simulink model "CAVE_MachE_sil_test"  (R2019b)
settings: configuration reference "ConfigSetDesktopFixedStep" (kept outside this file)
PreLoadFcn:
  | VSS_BICYCLE=Simulink.Variant('Dual=0');
  | VSS_DUAL=Simulink.Variant('Dual=1');
  | Dual=1;
  | load('DriveCycle2.mat')
PostLoadFcn:
  | if any(exist('dsrtsu_mdlpostloadfcn', 'file') ~= 0), dsrtsu_mdlpostloadfcn('Execute', bdroot); end
InitFcn:
  | , if any(exist('dsmpb_private', 'file') ~= 0), dsmpb_private('dsmpb_mdlclblib', 'Init', bdroot); end,
  | load('DriveCycle2.mat')
model workspace (MAT data in the model file):
  Gas = 0.383333333333
undefined symbols (not defined in the file or in its folder): AccelCmd, ActTqLF_Nm_, ActTqLR_Nm_, ActTqRF_Nm_, ActTqRR_Nm_, BattChargeLimitMaxPwr, BattChargeLimitSocBpts, BattChargeLimitTbl, BattChrgCapcty, BattDischargeLimitSocBpts, BattDischargeLimitTbl, BattDischargeMaxPwr, BattNumCellsParallel, BattNumCellsSeries, BattOpenVoltCapBpts, BattOpenVoltTbl, BattResistSocBpts, BattResistTbl, BattResistTempBpts, BrakeMaxPrs, BrakeMaxTrq, ChassisDistCg2FrontAxle, ChassisDistCg2RearAxle, ChassisVehMass, CltchCmd, CoastDown, DecelCmd, DiffRatio, DiscIntNeverNeededParam, EnvGravCnst, EnvPrs, EnvTemp, FuelSpecificGrav, GearCmd, h, InitStates, lgSw, limitedMCT, MCT, MtrEffSpdBpts, MtrEffTbl, MtrEffTrqBpts, MtrPwrMax, MtrTrqMax, pMCT, SteeringCmd, SupvsryCtrlRegenBrkCutOffTbl, SupvsryCtrlRegenSpdBpts, TestScnrioCycleNum, US06, VEH
libraries: VSIGenLib x39, simulink x27, etargetslib x24, CarMaker4SL x8, vehdynlibtire x8, vehdynlibsuspension x7, vehdynlibtirecommon x7, autolibutils x5, autolibshared x5, VsrLibWheel x4, sharedtransform x3, autolibbatterycommon x2
(part 3 of 11)

== system CAVE_MachE_sil_test/Vehicle Under Test/Vehicle/Rototest and ORNL Interface/RotoTrqPreprocess ==
  AxleTrqRaw : Inport
  Bus Selector1 : BusSelector  OutputSignals=ActTqLF_Nm_,ActTqRF_Nm_,ActTqLR_Nm_,ActTqRR_Nm_
  Compare To Constant : simulink/Logic and Bit Operations/Compare To Constant  relop=>=  const=-15  OutDataTypeStr=boolean
  Compare To Constant1 : simulink/Logic and Bit Operations/Compare To Constant  relop=<=  const=0  OutDataTypeStr=boolean
  Data Type Conversion{1..4} (4 alike) : DataTypeConversion  OutDataTypeStr=double
  FirstOrderFilterTau{,1..3} (4 alike) : VSIGenLib/FirstOrderFilterTau  SystemSampleTime=-1  Latency=0  AutoFrameSizeCalculation=off
  Ground : Ground
  Logical Operator : Logic  AllPortsSameDT=off  OutDataTypeStr=boolean
  ManualTrq_Nm : Constant  Value=0
  Mux : Mux
  Mux1 : Mux
  SatTrq : Saturate  UpperLimit=1000  LowerLimit=-1000
  Tau : Constant  Value=0.01
  TorqueIn : Switch  Criteria=u2 > Threshold
  "TorqueIn " : Switch  Criteria=u2 > Threshold
  AxleTrqRoto : Outport
  AxleTrqVeh : Outport  Port=2
  wires:
  Mux/1 -> AxleTrqRoto/1, TorqueIn/1
  ManualTrq_Nm/1 -> Mux1/4, Mux1/3, Mux1/2, Mux1/1
  Tau/1 -> FirstOrderFilterTau/2, FirstOrderFilterTau1/2, FirstOrderFilterTau2/2, FirstOrderFilterTau3/2
  Ground/1 -> "TorqueIn "/1
  Logical Operator/1 -> "TorqueIn "/2
  Data Type Conversion4/1 -> Mux/4  "RR"
  Data Type Conversion3/1 -> Mux/3  "LR"
  Mux1/1 -> TorqueIn/3
  [Switch] -> TorqueIn/2
  Bus Selector1/4 -> FirstOrderFilterTau3/1  "<ActTqRR_Nm_>"
  Compare To Constant/1 -> Logical Operator/1
  Bus Selector1/3 -> FirstOrderFilterTau2/1  "<ActTqLR_Nm_>"
  Bus Selector1/2 -> FirstOrderFilterTau1/1  "<ActTqRF_Nm_>"
  TorqueIn/1 -> SatTrq/1
  "TorqueIn "/1 -> AxleTrqVeh/1  "Trq"
  FirstOrderFilterTau1/1 -> Data Type Conversion2/1
  Data Type Conversion2/1 -> Mux/2  "RF"
  AxleTrqRaw/1 -> Bus Selector1/1
  FirstOrderFilterTau/1 -> Data Type Conversion1/1
  FirstOrderFilterTau3/1 -> Data Type Conversion4/1
  Bus Selector1/1 -> FirstOrderFilterTau/1  "<ActTqLF_Nm_>"
  Compare To Constant1/1 -> Logical Operator/2
  SatTrq/1 -> "TorqueIn "/3, Compare To Constant1/1, Compare To Constant/1
  FirstOrderFilterTau2/1 -> Data Type Conversion3/1
  Data Type Conversion1/1 -> Mux/1  "LF"

== system CAVE_MachE_sil_test/Vehicle Under Test/Vehicle/Rototest and ORNL Interface/Subsystem2 ==
  AxlTorq : Inport
  BusCreator1 : BusCreator  Inputs=16
  BusCreator2 : BusCreator  Inputs=16
  Constant : Constant  Value=0
  Constant1 : Constant  Value=0
  Demux : Demux  Outputs=16
  Terminator : Terminator
  Zero1 : Constant  Value=0
  Zero2 : Constant  Value=0
  Zero5 : Constant  Value=0
  BrakeUpd : Outport
  wires:
  Demux/9 -> BusCreator1/9  "Brake IF Trq_Reg_trg FL"
  Demux/6 -> BusCreator1/6  "Brake IF Trq_PB FR"
  Constant1/1 -> BusCreator2/1, BusCreator2/2  "Brake IF Trq_WB FL"
  Demux/14 -> BusCreator1/14  "Brake IF Trq_DriveSrc_trg d1"
  Zero2/1 -> BusCreator2/16, BusCreator2/15, BusCreator2/14, BusCreator2/13  "Brake IF Trq_DriveSrc_trg d3"
  Demux/11 -> BusCreator1/11  "Brake IF Trq_Reg_trg RL"
  Demux/15 -> BusCreator1/15  "Brake IF Trq_DriveSrc_trg d2"
  Demux/2 -> BusCreator1/2  "Brake IF Trq_WB FR"
  Demux/16 -> BusCreator1/16  "Brake IF Trq_DriveSrc_trg d3"
  Zero1/1 -> BusCreator2/12, BusCreator2/11, BusCreator2/10, BusCreator2/9  "Brake IF Trq_Reg_trg RR"
  Demux/4 -> BusCreator1/4  "Brake IF Trq_WB RR"
  Demux/3 -> BusCreator1/3  "Brake IF Trq_WB RL"
  Constant/1 -> BusCreator2/4, BusCreator2/3  "Brake IF Trq_WB RL"
  BusCreator1/1 -> BrakeUpd/1
  Demux/1 -> BusCreator1/1  "Brake IF Trq_WB FL"
  Demux/8 -> BusCreator1/8  "Brake IF Trq_PB RR"
  Demux/10 -> BusCreator1/10  "Brake IF Trq_Reg_trg FR"
  BusCreator2/1 -> Demux/1
  Demux/13 -> BusCreator1/13  "Brake IF Trq_DriveSrc_trg d0"
  Demux/5 -> BusCreator1/5  "Brake IF Trq_PB FL"
  Demux/7 -> BusCreator1/7  "Brake IF Trq_PB RL"
  Zero5/1 -> BusCreator2/8, BusCreator2/7, BusCreator2/6, BusCreator2/5  "Brake IF Trq_PB RR"
  Demux/12 -> BusCreator1/12  "Brake IF Trq_Reg_trg RR"
  AxlTorq/1 -> Terminator/1

== system CAVE_MachE_sil_test/Vehicle Under Test/Vehicle/Rototest and ORNL Interface/To Rototest with Band-Aid ==
  note: Torque Model: Low speed
      | Speed Model: Normal speed
  note: OutMode = 0 is Torque
      | OutMode = 1 is Speed
  note: Switch = 0 Overides
      | Switch = 1 Model
  SpeedCmd_rps : Inport
  AxleTrq_roto_Nm : Inport  Port=2
  BRAKE_PRESSED : Inport  Port=3
  Vehicle_Speed_kph : Inport  Port=4
  Band-Aid : Subsystem
  Demux : Demux
  Demux1 : Demux
  Demux2 : Demux
  Logging : Subsystem  Commented=on
  MasterSw : Constant
  Mode Override : Subsystem
  ModeOut : Switch  Criteria=u2 > Threshold
  ModeSwitch : MultiPortSwitch  DataPortOrder=Zero-based contiguous  Inputs=2  zeroidx=on
  Mux2 : Mux
  Mux4 : Mux
  Mux5 : Mux
  RateLimSpd : RateLimiter  RisingSlewLimit=500  FallingSlewLimit=-500  SampleTimeMode=inherited
  RotoTestEthTx : Subsystem  AncestorBlock=VSIGenLib/RotoTestEthTx
      mask Display:
      | color('white')
      | disp('RotTestEthTx')
      | port_label('input', 1, 'RefLF_NmORrpm')
      | port_label('input', 2, 'RefRF_NmORrpm')
      | port_label('input', 3, 'RefLR_NmORrpm')
      | port_label('input', 4, 'RefRR_NmORrpm')
      | port_label('input', 5, 'SqTrRR')
      | port_label('input', 6, 'SqTrLR')
      | port_label('input', 7, 'SqTrRF')
      | port_label('input', 8, 'SqTrLF')
      | port_label('input', 9, 'SystemActive')
      | port_label('output', 1, 'Status (bool)')
      | port_label('output', 2, 'Sent Bytes (int)')
  SatSpd : Saturate  UpperLimit=700  LowerLimit=0
  Scope : Scope
  Scope1 : Scope
  SpeedOut : Switch  Criteria=u2 > Threshold
  SystemActive : Constant  Value=0  OutDataTypeStr=uint8
  TrqSpd Override : Subsystem
  ZeroTorque : Constant  Value=0  OutDataTypeStr=uint8
  rads2rpm : Gain  Gain=9.5492965964254
  Out1 : Outport
  tag scope: Switch=global
  wires:
  Mux4/1 -> ModeSwitch/2
  Demux/3 -> Mux2/3  "LRIn"
  Demux1/4 -> RotoTestEthTx/4(RefRR_NmORrpm)
  Demux/2 -> Mux2/2  "RFIn"
  MasterSw/1 -> [Switch]
  TrqSpd Override/1(Ovr) -> SpeedOut/3
  ZeroTorque/1 -> Mux4/2, Mux4/3, Mux4/4, Mux4/1
  Demux/1 -> Mux2/1  "LFIn"
  SpeedOut/1 -> RateLimSpd/1
  RateLimSpd/1 -> SatSpd/1
  rads2rpm/1 -> Demux/1
  ModeSwitch/1 -> Demux1/1
  Demux/4 -> Mux2/4  "RRIn"
  Band-Aid/1(OutMode) -> Mux5/4, Mux5/3, Mux5/2, Mux5/1, ModeSwitch/1
  ModeOut/1 -> Demux2/1
  [Switch] -> SpeedOut/2
  SatSpd/1 -> Scope1/1, ModeSwitch/3  "Spd"
  [Switch] -> ModeOut/2
  Mux5/1 -> ModeOut/1
  Demux2/1 -> RotoTestEthTx/5(SpTqRR)
  Demux1/3 -> RotoTestEthTx/3(RefLR_NmORrpm)
  Demux2/3 -> RotoTestEthTx/7(SpTqRF)
  Demux2/2 -> RotoTestEthTx/6(SpTqLR)
  SystemActive/1 -> RotoTestEthTx/9(SystemActive)
  RotoTestEthTx/1(Output) -> Out1/1  "ByteSend"
  Demux1/1 -> Scope/1, RotoTestEthTx/1(RefLF_NmORrpm)
  Demux1/2 -> RotoTestEthTx/2(RefRF_NmORrpm)
  Demux2/4 -> RotoTestEthTx/8(SpTqLF)
  SpeedCmd_rps/1 -> rads2rpm/1
  Mode Override/1(Ovr) -> ModeOut/3
  AxleTrq_roto_Nm/1 -> Band-Aid/2(InTrq_Nm)
  Mux2/1 -> Band-Aid/1(InSpd_rpm)
  Band-Aid/2(OutSpd_rpm) -> SpeedOut/1
  BRAKE_PRESSED/1 -> Band-Aid/3(BRAKE_PRESSED)
  Vehicle_Speed_kph/1 -> Band-Aid/4(VehSpd_kph)

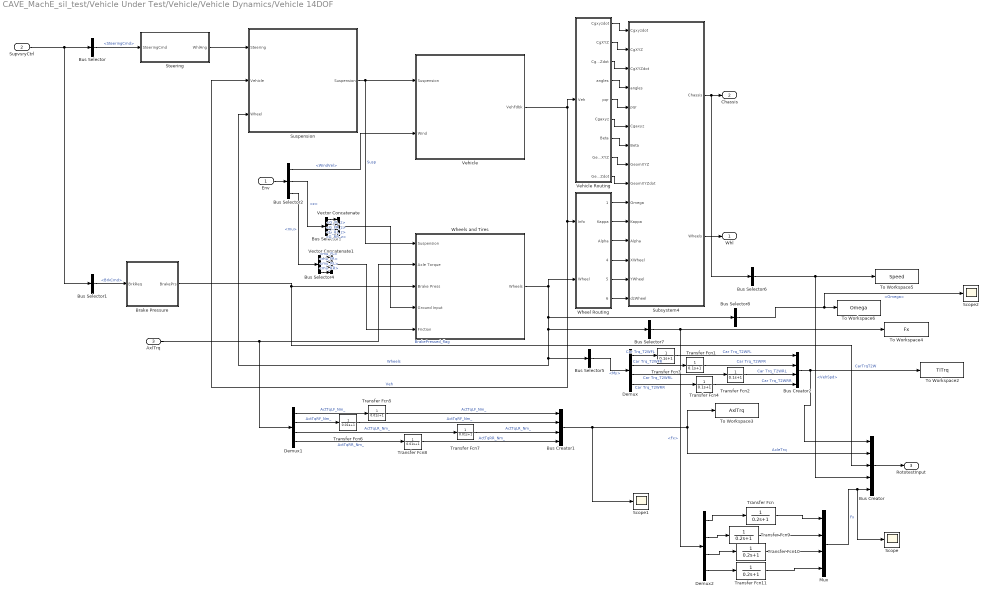
== system CAVE_MachE_sil_test/Vehicle Under Test/Vehicle/Vehicle Dynamics/Vehicle 14DOF ==
  Env : Inport
  SupvsryCtrl : Inport  Port=2
  AxlTrq : Inport  Port=3
  Brake Pressure : Subsystem
  Bus Creator : BusCreator  Inputs=5
  Bus Creator1 : BusCreator  Inputs=ActTqLF_Nm_,ActTqRF_Nm_,ActTqLR_Nm_,ActTqRR_Nm_
  Bus Creator2 : BusCreator  Inputs=Car Trq_T2WFL,Car Trq_T2WFR,Car Trq_T2WRL,Car Trq_T2WRR
  Bus Selector : BusSelector  OutputSignals=SteeringCmd
  Bus Selector1 : BusSelector  OutputSignals=BrkCmd
  Bus Selector2 : BusSelector  OutputSignals=WindVel,GndBus.z,GndBus.mu
  Bus Selector3 : BusSelector  OutputSignals=G_FL_z,G_FR_z,G_RL_z,G_RR_z
  Bus Selector4 : BusSelector  OutputSignals=mu_FL,mu_FR,mu_RL,mu_RR
  Bus Selector5 : BusSelector  OutputSignals=TireFrame.My
  Bus Selector6 : BusSelector  OutputSignals=VehSpd
  Bus Selector7 : BusSelector  OutputSignals=TireFrame.Fx
  Bus Selector8 : BusSelector  OutputSignals=TireFrame.Omega
  Demux : Demux
  Demux1 : Demux
  Demux2 : Demux
  Mux : Mux
  Scope : Scope
  Scope1 : Scope
  Scope2 : Scope
  Steering : Subsystem
  Subsystem4 : Subsystem
  Suspension : Subsystem  VariantControlMode=Label  Variant=on  LabelModeActiveChoice=3
      mask Display:
      | switch str2num(get_param(gcb,'ActiveVariant'))
      |     case 1
      |         image('suspdw.png');
      |     case 2
      |         image([imread('suspindmap.png');imread('suspsamap.png')]);
      |     case 3
      |          image([imread('suspmacp.png');imread('suspsacoil.png')]);
      |     case 4
      |          image('suspmacp.png');
      |     case 5
      |          image('suspindmap.png');
      | end
  To Workspace2 : ToWorkspace  VariableName=TiTrq  SampleTime=-1
      settings: Save2DSignal=2-D array (concatenate along first dimension)
  To Workspace3 : ToWorkspace  VariableName=AxlTrq  SampleTime=-1
      settings: Save2DSignal=2-D array (concatenate along first dimension)
  To Workspace4 : ToWorkspace  VariableName=Fx  SampleTime=-1
      settings: Save2DSignal=2-D array (concatenate along first dimension)
  To Workspace5 : ToWorkspace  VariableName=Speed  SampleTime=-1
      settings: Save2DSignal=2-D array (concatenate along first dimension)
  To Workspace6 : ToWorkspace  VariableName=Omega  SampleTime=-1
      settings: Save2DSignal=2-D array (concatenate along first dimension)
  Transfer Fcn{,9..11} (4 alike) : TransferFcn  Denominator=[0.2 1]
  Transfer Fcn{1..4} (4 alike) : TransferFcn  Denominator=[0.1 1]
  Transfer Fcn{5..8} (4 alike) : TransferFcn  Denominator=[0.01 1]
  Vector Concatenate : Concatenate  NumInputs=4
  Vector Concatenate1 : Concatenate  NumInputs=4
  Vehicle : Subsystem
      mask Display: image('6dofcar.png');
  Vehicle Routing : Subsystem
  Wheel Routing : Subsystem
  Wheels and Tires : Subsystem
      mask Display: image('wheel3dof.png')
  Whl : Outport
  Chassis : Outport  Port=2
  RototestInput : Outport  Port=3
  wires:
  Vehicle Routing/9(GeomXYZdot) -> Subsystem4/9(GeomXYZdot)
  Vehicle Routing/8(GeomXYZ) -> Subsystem4/8(GeomXYZ)
  Vehicle Routing/1(Cgxyzdot) -> Subsystem4/1(Cgxyzdot)
  Vehicle Routing/5(pqr) -> Subsystem4/5(pqr)
  Vehicle Routing/4(angles) -> Subsystem4/4(angles)
  Vehicle Routing/3(CgXYZdot) -> Subsystem4/3(CgXYZdot)
  Vehicle Routing/7(Beta) -> Subsystem4/7(Beta)
  Wheels and Tires/1(Wheels) -> Wheel Routing/2(Wheel), Bus Selector7/1, Bus Selector5/1, Suspension/3(Wheel), Bus Selector8/1  "Wheels"
  Vehicle Routing/2(CgXYZ) -> Subsystem4/2(CgXYZ)
  Vehicle/1(VehFdbk) -> Suspension/2(Vehicle), Wheel Routing/1(Info), Vehicle Routing/1(Veh)  "Veh"
  Suspension/1(Suspension) -> Vehicle/1(Suspension), Wheels and Tires/1(Suspension)  "Susp"
  Bus Selector2/1 -> Vehicle/2(Wind)  "<WindVel>"
  Steering/1(WhlAng) -> Suspension/1(Steering)
  Bus Selector/1 -> Steering/1(SteeringCmd)  "<SteeringCmd>"
  SupvsryCtrl/1 -> Bus Selector/1, Bus Selector1/1
  Bus Selector1/1 -> Brake Pressure/1(BrkReq)  "<BrkCmd>"
  Env/1 -> Bus Selector2/1
  Vehicle Routing/6(Cgaxyz) -> Subsystem4/6(Cgaxyz)
  Wheel Routing/1(Omega) -> Subsystem4/10(Omega)
  Wheel Routing/3(Alpha) -> Subsystem4/12(Alpha)
  Wheel Routing/4(XWheel) -> Subsystem4/13(XWheel)
  Wheel Routing/2(Kappa) -> Subsystem4/11(Kappa)
  Wheel Routing/5(YWheel) -> Subsystem4/14(YWheel)
  Wheel Routing/6(ZWheel) -> Subsystem4/15(dzWheel)
  Subsystem4/2(Wheels) -> Whl/1
  AxlTrq/1 -> Demux1/1, Wheels and Tires/2(Axle Torque)
  Bus Selector2/2 -> Bus Selector3/1  "<z>"
  Bus Selector3/1 -> Vector Concatenate/1  "<G_FL_z>"
  Bus Selector3/2 -> Vector Concatenate/2  "<G_FR_z>"
  Bus Selector3/3 -> Vector Concatenate/3  "<G_RL_z>"
  Bus Selector3/4 -> Vector Concatenate/4  "<G_RR_z>"
  Vector Concatenate/1 -> Wheels and Tires/4(Ground Input)
  Bus Selector4/4 -> Vector Concatenate1/4  "<mu_RR>"
  Bus Selector2/3 -> Bus Selector4/1  "<mu>"
  Bus Selector4/3 -> Vector Concatenate1/3  "<mu_RL>"
  Bus Selector4/2 -> Vector Concatenate1/2  "<mu_FR>"
  Bus Selector4/1 -> Vector Concatenate1/1  "<mu_FL>"
  Vector Concatenate1/1 -> Wheels and Tires/5(Friction)
  Demux/3 -> Transfer Fcn2/1  "Car Trq_T2WRL"
  Bus Selector6/1 -> Bus Creator/4, To Workspace5/1  "<VehSpd>"
  Brake Pressure/1(BrakePrs) -> Bus Creator/3, Wheels and Tires/3(Brake Press)  "BrakePressed_flag"
  Demux/2 -> Transfer Fcn1/1  "Car Trq_T2WFR"
  Demux1/1 -> Transfer Fcn5/1  "ActTqLF_Nm_"
  Demux1/4 -> Transfer Fcn8/1  "ActTqRR_Nm_"
  Demux1/3 -> Transfer Fcn7/1  "ActTqLR_Nm_"
  Demux/4 -> Transfer Fcn4/1  "Car Trq_T2WRR"
  Bus Creator1/1 -> Scope1/1, Bus Creator/2, To Workspace3/1  "AxleTrq"
  Demux1/2 -> Transfer Fcn6/1  "ActTqRF_Nm_"
  Bus Creator2/1 -> Bus Creator/1, To Workspace2/1  "CarTrqT2W"
  Demux/1 -> Transfer Fcn3/1  "Car Trq_T2WFL"
  Bus Selector5/1 -> Demux/1  "<My>"
  Subsystem4/1(Chassis) -> Bus Selector6/1, Chassis/1
  Bus Selector7/1 -> Demux2/1, To Workspace4/1  "<Fx>"
  Bus Selector8/1 -> Scope2/1, To Workspace6/1  "<Omega>"
  Bus Creator/1 -> RototestInput/1
  Transfer Fcn3/1 -> Bus Creator2/1  "Car Trq_T2WFL"
  Transfer Fcn1/1 -> Bus Creator2/2  "Car Trq_T2WFR"
  Transfer Fcn2/1 -> Bus Creator2/3  "Car Trq_T2WRL"
  Transfer Fcn4/1 -> Bus Creator2/4  "Car Trq_T2WRR"
  Transfer Fcn5/1 -> Bus Creator1/1  "ActTqLF_Nm_"
  Transfer Fcn6/1 -> Bus Creator1/2  "ActTqRF_Nm_"
  Transfer Fcn7/1 -> Bus Creator1/3  "ActTqLR_Nm_"
  Transfer Fcn8/1 -> Bus Creator1/4  "ActTqRR_Nm_"
  Demux2/1 -> Transfer Fcn/1
  Transfer Fcn/1 -> Mux/1
  Demux2/2 -> Transfer Fcn9/1
  Transfer Fcn9/1 -> Mux/2
  Demux2/3 -> Transfer Fcn10/1
  Demux2/4 -> Transfer Fcn11/1
  Transfer Fcn10/1 -> Mux/3
  Transfer Fcn11/1 -> Mux/4
  Mux/1 -> Scope/1, Bus Creator/5  "Fx"

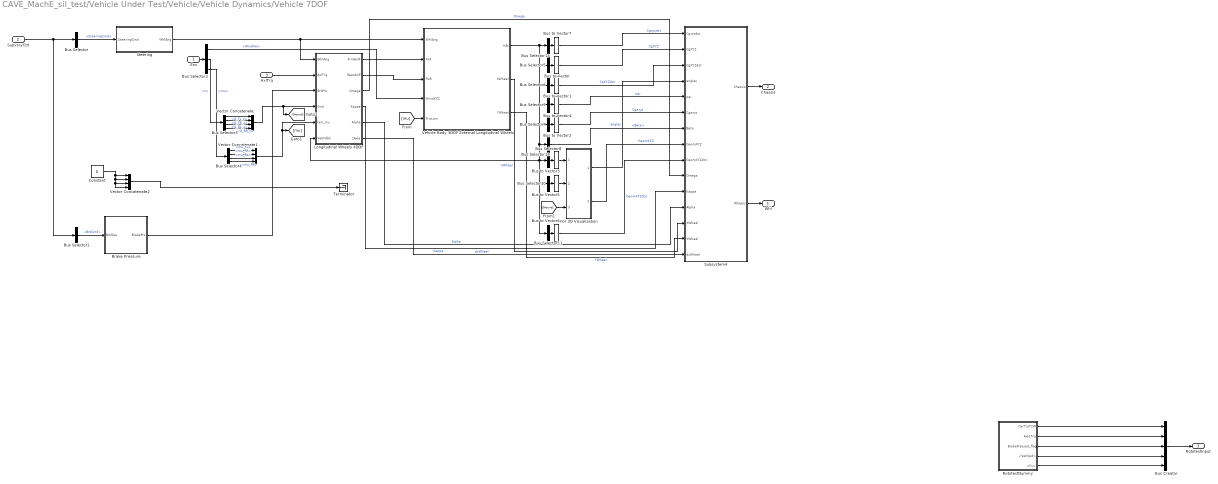
== system CAVE_MachE_sil_test/Vehicle Under Test/Vehicle/Vehicle Dynamics/Vehicle 7DOF ==
  Env : Inport
  SupvsryCtrl : Inport  Port=2
  AxlTrq : Inport  Port=3
  Brake Pressure : Subsystem
  Bus Creator : BusCreator  Inputs=5
  Bus Selector : BusSelector  OutputSignals=SteeringCmd
  Bus Selector1 : BusSelector  OutputSignals=BrkCmd
  Bus Selector10 : BusSelector  OutputSignals=InertFrm.Geom.Disp.X,InertFrm.Geom.Disp.Y,InertFrm.Geom.Disp.Z  OutputAsBus=on
  Bus Selector11 : BusSelector  OutputSignals=InertFrm.Geom.Vel.Xdot,InertFrm.Geom.Vel.Ydot,InertFrm.Geom.Vel.Zdot  OutputAsBus=on
  Bus Selector12 : BusSelector  OutputSignals=BdyFrm.Geom.Ang.Beta
  Bus Selector13 : BusSelector  OutputSignals=BdyFrm.Cg.Vel.xdot,BdyFrm.Cg.Vel.ydot,BdyFrm.Cg.Vel.zdot  OutputAsBus=on
  Bus Selector2 : BusSelector  OutputSignals=WindVel,GndBus.z,GndBus.mu
  Bus Selector3 : BusSelector  OutputSignals=G_FL_z,G_FR_z,G_RL_z,G_RR_z
  Bus Selector4 : BusSelector  OutputSignals=mu_FL,mu_FR,mu_RL,mu_RR
  Bus Selector5 : BusSelector  OutputSignals=InertFrm.Cg.Disp.X,InertFrm.Cg.Disp.Y,InertFrm.Cg.Disp.Z  OutputAsBus=on
  Bus Selector6 : BusSelector  OutputSignals=InertFrm.Cg.Vel.Xdot,InertFrm.Cg.Vel.Ydot,InertFrm.Cg.Vel.Zdot  OutputAsBus=on
  Bus Selector7 : BusSelector  OutputSignals=BdyFrm.Cg.Acc.ax,BdyFrm.Cg.Acc.ay,BdyFrm.Cg.Acc.az  OutputAsBus=on
  Bus Selector8 : BusSelector  OutputSignals=InertFrm.Cg.Ang.phi,InertFrm.Cg.Ang.theta,InertFrm.Cg.Ang.psi  OutputAsBus=on
  Bus Selector9 : BusSelector  OutputSignals=BdyFrm.Cg.AngVel.p,BdyFrm.Cg.AngVel.q,BdyFrm.Cg.AngVel.r  OutputAsBus=on
  Bus to Vector{,1..7} (8 alike) : BusToVector
  Constant : Constant  Value=0
  For 3D Visualization : MATLAB Function  TreatAsAtomicUnit=on  mask{trackW=1.9, wheelB=ChassisDistCg2FrontAxle+ChassisDistCg2RearAxle}
      mask prompts: trackW "Vehicle track width, trackW [m]:"; wheelB "Vehicle wheelbase, wheelB [m]:"
      mask help: This block converts wheel ground height information into estimates of vehicle pitch, roll angles and vertical height in order to help in the visualization 3DOF based simulations with changes in terrain. Note that the resulting signals are only used as a visualization aid and do not account for the physical affects of the vehicle interacting with variable terrain or changes in orientation.
  Longitudinal Wheels 4DOF : Subsystem  VariantControl=1
      settings: AttributesFormatString=%<wheelMode>
  RototestDummy : Subsystem
  Steering : Subsystem
  Subsystem4 : Subsystem
  Terminator : Terminator
  Vector Concatenate : Concatenate  NumInputs=4
  Vector Concatenate1 : Concatenate  NumInputs=4
  Vector Concatenate2 : Concatenate  NumInputs=4
  Vehicle Body 3DOF External Longitudinal Wheels : Subsystem  VariantControlMode=Label  Variant=on  VariantControl=Variant1  LabelModeActiveChoice=1
      settings: AttributesFormatString=%<trackMode>
  Whl : Outport
  Chassis : Outport  Port=2
  RototestInput : Outport  Port=3
  wires:
  Bus Selector2/1 -> Vehicle Body 3DOF External Longitudinal Wheels/4(WindXYZ)  "<WindVel>"
  Bus Selector/1 -> Steering/1(SteeringCmd)  "<SteeringCmd>"
  SupvsryCtrl/1 -> Bus Selector/1, Bus Selector1/1
  Bus Selector1/1 -> Brake Pressure/1(BrkReq)  "<BrkCmd>"
  Env/1 -> Bus Selector2/1
  Subsystem4/2(Wheels) -> Whl/1
  Subsystem4/1(Chassis) -> Chassis/1
  Bus Selector2/2 -> Bus Selector3/1  "<z>"
  Bus Selector3/1 -> Vector Concatenate/1  "<G_FL_z>"
  Bus Selector3/2 -> Vector Concatenate/2  "<G_FR_z>"
  Bus Selector3/3 -> Vector Concatenate/3  "<G_RL_z>"
  Bus Selector3/4 -> Vector Concatenate/4  "<G_RR_z>"
  Bus Selector4/4 -> Vector Concatenate1/4  "<mu_RR>"
  Bus Selector2/3 -> Bus Selector4/1  "<mu>"
  Bus Selector4/3 -> Vector Concatenate1/3  "<mu_RL>"
  Bus Selector4/2 -> Vector Concatenate1/2  "<mu_FR>"
  Bus Selector4/1 -> Vector Concatenate1/1  "<mu_FL>"
  Vector Concatenate2/1 -> Terminator/1
  Constant/1 -> Vector Concatenate2/4, Vector Concatenate2/3, Vector Concatenate2/2, Vector Concatenate2/1
  Bus to Vector2/1 -> Subsystem4/6(Cgaxyz)  "Cgaxyz"
  Bus Selector8/1 -> Bus to Vector3/1
  Bus to Vector5/1 -> For 3D Visualization/2(GemoXYZIn)
  Bus Selector12/1 -> Subsystem4/7(Beta)  "<Beta>"
  Bus Selector5/1 -> Bus to Vector/1
  For 3D Visualization/1(angles) -> Subsystem4/4(angles)  "angles"
  For 3D Visualization/2(GeomXYZ) -> Subsystem4/8(GeomXYZ)  "GeomXYZ"
  Bus to Vector6/1 -> Subsystem4/9(GeomXYZdot)  "GeomXYZdot"
  Bus Selector13/1 -> Bus to Vector7/1
  Bus to Vector7/1 -> Subsystem4/1(Cgxyzdot)  "Cgxyzdot"
  Bus Selector10/1 -> Bus to Vector5/1
  Longitudinal Wheels 4DOF/1(FrntAxlF) -> Vehicle Body 3DOF External Longitudinal Wheels/2("FwF ")
  Bus Selector11/1 -> Bus to Vector6/1
  Bus Selector9/1 -> Bus to Vector4/1
  [mu] -> Vehicle Body 3DOF External Longitudinal Wheels/5(Friction)
  Longitudinal Wheels 4DOF/2(RearAxlF) -> Vehicle Body 3DOF External Longitudinal Wheels/3("FwR ")
  Bus to Vector4/1 -> Subsystem4/5(pqr)  "pqr"
  Vehicle Body 3DOF External Longitudinal Wheels/3(" YWheel") -> Subsystem4/14(YWheel)  "YWheel"
  Vector Concatenate/1 -> Longitudinal Wheels 4DOF/4(Gnd), [Ground]
  Bus to Vector/1 -> Subsystem4/2(CgXYZ)  "CgXYZ"
  AxlTrq/1 -> Longitudinal Wheels 4DOF/2(AxlTrq)
  Vehicle Body 3DOF External Longitudinal Wheels/1(" Info") -> Bus Selector13/1, Bus Selector11/1, Bus Selector10/1, Longitudinal Wheels 4DOF/6(VehFdbk), Bus Selector8/1, Bus Selector12/1, Bus Selector7/1, Bus Selector9/1, Bus Selector6/1, Bus Selector5/1
  [Ground] -> For 3D Visualization/3(GroundZ)
  Bus to Vector1/1 -> Subsystem4/3(CgXYZdot)  "CgXYZdot"
  Bus to Vector3/1 -> For 3D Visualization/1(angleIn)
  Longitudinal Wheels 4DOF/5(Alpha) -> Subsystem4/12(Alpha)  "Alpha"
  Vector Concatenate1/1 -> Longitudinal Wheels 4DOF/5(lam_mu), [mu]
  Bus Selector6/1 -> Bus to Vector1/1
  Brake Pressure/1(BrakePrs) -> Longitudinal Wheels 4DOF/3(BrkPrs)
  Vehicle Body 3DOF External Longitudinal Wheels/2(" XWheel") -> Subsystem4/13(XWheel)  "XWheel"
  Longitudinal Wheels 4DOF/4(Kappa) -> Subsystem4/11(Kappa)  "Kappa"
  Steering/1(WhlAng) -> Longitudinal Wheels 4DOF/1(WhlAng), Vehicle Body 3DOF External Longitudinal Wheels/1(WhlAng)
  Longitudinal Wheels 4DOF/6(zAxle) -> Subsystem4/15(dzWheel)  "dzWheel"
  Bus Selector7/1 -> Bus to Vector2/1
  Longitudinal Wheels 4DOF/3(Omega) -> Subsystem4/10(Omega)  "Omega"
  Bus Creator/1 -> RototestInput/1
  RototestDummy/1(CarTrqT2W) -> Bus Creator/1
  RototestDummy/2(AxleTrq) -> Bus Creator/2
  RototestDummy/3(BrakePressed_flag) -> Bus Creator/3
  RototestDummy/4(<VehSpd>) -> Bus Creator/4
  RototestDummy/5(<Fx>) -> Bus Creator/5

== system CAVE_MachE_sil_test/Vehicle Under Test/Vehicle/Vehicle Dynamics/Vehicle Longitudinal ==
  Env : Inport
  SupvsryCtrl : Inport  Port=2
  AxlTrq : Inport  Port=3
  Brake Pressure : Subsystem
  Bus Creator : BusCreator  Inputs=5
  Bus Selector1 : BusSelector  OutputSignals=BrkCmd
  Bus Selector2 : BusSelector  OutputSignals=RoadGrade,WindVel,GndBus.z,GndBus.mu
  Bus Selector3 : BusSelector  OutputSignals=G_FL_z,G_FR_z,G_RL_z,G_RR_z
  Bus Selector4 : BusSelector  OutputSignals=mu_FL,mu_FR,mu_RL,mu_RR
  Constant : Constant  Value=0
  Longitudinal Wheels : Subsystem  AncestorBlock=LibWheels/Longitudinal Wheels and Brakes
  RototestDummy : Subsystem
  Selector : Selector  InputPortWidth=3  IndexOptions=Index vector (dialog)  Indices=1  OutputSizes=1
  Terminator : Terminator
  Terminator1 : Terminator
  Vector Concatenate : Concatenate  NumInputs=4
  Vector Concatenate1 : Concatenate  NumInputs=4
  Vector Concatenate2 : Concatenate  NumInputs=4
  Vehicle Body : Subsystem
  Whl : Outport
  Chassis : Outport  Port=2
  RototestInput : Outport  Port=3
  wires:
  Vehicle Body/1(Chassis) -> Chassis/1
  Longitudinal Wheels/1(Whl) -> Whl/1
  Bus Selector4/1 -> Vector Concatenate1/1  "<mu_FL>"
  Bus Selector2/4 -> Bus Selector4/1  "<mu>"
  Vector Concatenate1/1 -> Terminator1/1
  Brake Pressure/1(BrakePrs) -> Longitudinal Wheels/1(BrkPrs)
  Bus Selector4/2 -> Vector Concatenate1/2  "<mu_FR>"
  Bus Selector3/1 -> Vector Concatenate/1  "<G_FL_z>"
  Bus Selector3/4 -> Vector Concatenate/4  "<G_RR_z>"
  Bus Selector2/3 -> Bus Selector3/1  "<z>"
  Env/1 -> Bus Selector2/1
  Vector Concatenate/1 -> Terminator/1
  Bus Selector4/3 -> Vector Concatenate1/3  "<mu_RL>"
  Bus Selector3/2 -> Vector Concatenate/2  "<G_FR_z>"
  SupvsryCtrl/1 -> Bus Selector1/1
  Constant/1 -> Vector Concatenate2/4, Vector Concatenate2/3, Vector Concatenate2/2, Vector Concatenate2/1
  Bus Selector4/4 -> Vector Concatenate1/4  "<mu_RR>"
  Bus Selector1/1 -> Brake Pressure/1(BrkReq)  "<BrkCmd>"
  Bus Selector3/3 -> Vector Concatenate/3  "<G_RL_z>"
  AxlTrq/1 -> Longitudinal Wheels/2(AxleTorq)
  Bus Selector2/2 -> Selector/1  "<WindVel>"
  Bus Selector2/1 -> Vehicle Body/1(RoadGrade)  "<RoadGrade>"
  Selector/1 -> Vehicle Body/2(WindX)
  Bus Creator/1 -> RototestInput/1
  RototestDummy/5(<Fx>) -> Bus Creator/5
  RototestDummy/4(<VehSpd>) -> Bus Creator/4
  RototestDummy/3(BrakePressed_flag) -> Bus Creator/3
  RototestDummy/2(AxleTrq) -> Bus Creator/2
  RototestDummy/1(CarTrqT2W) -> Bus Creator/1
  connections:
  Longitudinal Wheels/RConn2 -- Vehicle Body/LConn2
  Vehicle Body/LConn1 -- Longitudinal Wheels/RConn1

== system CAVE_MachE_sil_test/Vehicle Under Test/Vehicle/Battery/Battery/Lithium Ion Battery Pack1 ==
  note: Info
  BattCurr : Inport  Unit=A
  BattTemp : Inport  Port=2  Unit=K
  Datasheet Battery Internal : Subsystem  AncestorBlock=autolibbatterycommon/Datasheet Battery Internal
  Info Bus : autolibbatterycommon/Info  RefBlkName='autolibdatasheetbattery/Datasheet Battery'
      settings: SourceProductName=Powertrain Blockset  SourceProductBaseCode=PW
  Output Passthrough : autolibbatterycommon/Output Passthrough  SystemSampleTime=-1  Latency=0  AutoFrameSizeCalculation=off
      settings: SourceProductName=Powertrain Blockset  SourceProductBaseCode=PW
  Info : Outport  VectorParamsAs1DForOutWhenUnconnected=off
  BattVolt : Outport  Port=2  Unit=V  VectorParamsAs1DForOutWhenUnconnected=off
  wires:
  [BattPwrLoss] -> Info Bus/5
  Output Passthrough/1 -> BattVolt/1, [BattVolt]
  [BattVolt] -> Info Bus/4
  Datasheet Battery Internal/1(LdCurrFeed) -> [LdCurrFeed]
  [LdCurrFeed] -> Info Bus/3
  Datasheet Battery Internal/5(BattPwrLoss) -> [BattPwrLoss]
  Datasheet Battery Internal/2(OutVoltUnfilt) -> Output Passthrough/1
  Datasheet Battery Internal/3(LdAmpHr) -> [LdAmpHr]
  Datasheet Battery Internal/4(BattSoc) -> [BattSoc]
  BattTemp/1 -> Datasheet Battery Internal/2(BattTemp)
  BattCurr/1 -> Datasheet Battery Internal/1(BattCurr)
  Info Bus/1 -> Info/1
  [BattSoc] -> Info Bus/2
  [LdAmpHr] -> Info Bus/1

== system CAVE_MachE_sil_test/Vehicle Under Test/Vehicle/Driver and Drive Cycle/Driver and PI with FF Control/Vehicle Speed Controller ==
  note: ToDo: Maybe do something clever with FF and Brake, or maybe not.
      | Bleed FF based on refspd derivative
  RefSpd : Inport
  VehicleSpeed : Inport  Port=2
  Compare To Constant1 : simulink/Logic and Bit Operations/Compare To Constant  relop=<=  const=0.1  OutDataTypeStr=boolean  ZeroCross=off
  Compare To Constant3 : simulink/Logic and Bit Operations/Compare To Constant  relop=<=  const=0  OutDataTypeStr=boolean  ZeroCross=off
  Constant : Constant  Value=0
  Constant1 : Constant  Value=0
  Feedforward : Lookup_n-D  NumberOfTableDimensions=1  BreakpointsForDimension1="[0 10    20    30    40    50    60    70    80    90   100   110   120   130   140   150   160]"  Table="[0\t3.5\t12.5\t16\t20\t21\t22\t24.5\t26\t29.5\t32\t33\t34\t36\t37\t38\t39]"  ExtrapMethod=Clip  InternalRulePriority=Speed  RndMeth=Simplest  InputSameDT=on
  Feedforward1 : Lookup_n-D  NumberOfTableDimensions=1  BreakpointsForDimension1="[0 10    20    30    40    50    60    70    80    90   100   110   120   130   140   150   160]"  Table="[0 2.6021    4.7790    6.8575    8.1555    9.4176   10.7914   12.3245   14.1570   15.9699   17.4605   19.0355   21.3079   22.8407   25.3373   26.9453   28.6975]"  ExtrapMethod=Clip  InternalRulePriority=Speed  RndMeth=Simplest  InputSameDT=on
  FeedforwardGain : Gain
  Gain : Gain  Gain=-1
  Ki : Gain  Gain=2
  Kp : Gain  Gain=10
  Limits [-50,50] : Integrator  ExternalReset=either  LimitOutput=on  UpperSaturationLimit=50  LowerSaturationLimit=-50
  Lowpass Filter : TransferFcn  Denominator=[.02 1]
  Min threshold for Brake switch : Constant  Value=0
  Product1 : Product  RndMeth=Zero
  Proportional Gain Scheduling : Lookup_n-D  NumberOfTableDimensions=1  BreakpointsForDimension1=[ 0 30 70]  IndexSearchMethod=Linear search  BeginIndexSearchUsingPreviousIndexResult=on  Table=[1 1 1]  ExtrapMethod=Clip  UseLastTableValue=on  RndMeth=Simplest  InputSameDT=on
  Relational Operator : RelationalOperator  Operator=>  OutDataTypeStr=boolean  RndMeth=Nearest
  Sum : Sum  Inputs=|+-
  Sum1 : Sum  Inputs=+++
  Switch{1..4} (4 alike) : Switch  Criteria=u2 > Threshold
  standstill brake [0,100] : Constant  Value=50
  AcceleratorPedalPos : Outport  VectorParamsAs1DForOutWhenUnconnected=off
  BrakePedalPos : Outport  Port=2  VectorParamsAs1DForOutWhenUnconnected=off
  BrakeSwitch : Outport  Port=3  VectorParamsAs1DForOutWhenUnconnected=off
  wires:
  Kp/1 -> Product1/1
  Min threshold for Brake switch/1 -> Relational Operator/2
  Switch1/1 -> Switch3/3  "AcceleratorPedalPosPre_pct"
  RefSpd/1 -> Feedforward1/1, Compare To Constant1/1, Compare To Constant3/1, Sum/1  "RefSpd"
  Sum/1 -> Kp/1, Ki/1  "SpdErr"
  Limits [-50,50]/1 -> Sum1/1  "Driver_IntTerm_pct"
  VehicleSpeed/1 -> Proportional Gain Scheduling/1, Lowpass Filter/1
  Switch2/1 -> Switch4/3, Relational Operator/1  "BrakePedalPosPre_pct"
  Lowpass Filter/1 -> Sum/2  "VS_Flt"
  Relational Operator/1 -> BrakeSwitch/1  "BrakeSwitch"
  Sum1/1 -> Gain/1, Switch1/1, Switch1/2  "Driver_TotCmdPreLim_pct"
  Ki/1 -> Limits [-50,50]/1
  Constant1/1 -> Switch2/3, Switch1/3
  Gain/1 -> Switch2/1, Switch2/2
  Compare To Constant3/1 -> Limits [-50,50]/2
  Compare To Constant1/1 -> Switch3/2, Switch4/2
  Switch3/1 -> AcceleratorPedalPos/1  "AcceleratorPedalPos_pct"
  Constant/1 -> Switch3/1
  standstill brake [0,100]/1 -> Switch4/1
  Switch4/1 -> BrakePedalPos/1  "BrakePedalPos_pct"
  Proportional Gain Scheduling/1 -> Product1/2
  Product1/1 -> Sum1/2  "Driver_PropTerm_pct"
  Feedforward1/1 -> FeedforwardGain/1
  FeedforwardGain/1 -> Sum1/3  "Driver_FdfwdTerm_pct"

== system CAVE_MachE_sil_test/Vehicle Under Test/Vehicle/Front Wheel Drive/Ideal Diff/Power Bus ==
  DriveshftTrq : Inport
  Speed : Inport  Port=2
  Bus Creator : BusCreator  Inputs=1
  Bus Creator5 : BusCreator  Inputs=2
  Bus Creator6 : BusCreator  Inputs=3
  Bus Creator7 : BusCreator  Inputs=1
  Constant : Constant  Value=0
  Constant1 : Constant  Value=0
  Constant2 : Constant  Value=0
  Demux : Demux  Outputs=3
  Power Accounting Bus Creator : autolibpowerinfoutils/Power Accounting Bus Creator  AssctBlkSelPopup=Parent reference block  RefBlkName='autolibshareddiff/Open Differential'  PwrTrnsfrdCheckBox=on  PwrNotTrnsfrdCheckBox=on  PwrStoredCheckBox=on  aMode=aMode
      settings: SourceProductName=Powertrain Blockset  SourceProductBaseCode=PW
  Signal Specification5 : SignalSpecification  Unit=W
  Transferred Power : Product
  Vector Concatenate : Concatenate  NumInputs=3
  PwrInfo : Outport
  wires:
  Bus Creator/1 -> Power Accounting Bus Creator/1
  Power Accounting Bus Creator/1 -> PwrInfo/1  "PwrInfo"
  Bus Creator5/1 -> Power Accounting Bus Creator/2
  Bus Creator6/1 -> Bus Creator/1  "PwrTrnsfrd"
  Transferred Power/1 -> Signal Specification5/1
  Signal Specification5/1 -> Vector Concatenate/3, Vector Concatenate/2, Vector Concatenate/1  "PwrDriveshft"
  Constant/1 -> Bus Creator5/1  "PwrMechLoss"
  Demux/3 -> Bus Creator6/3  "PwrAxl2"
  DriveshftTrq/1 -> Transferred Power/1
  Bus Creator7/1 -> Power Accounting Bus Creator/3
  Demux/2 -> Bus Creator6/2  "PwrAxl1"
  Demux/1 -> Bus Creator6/1  "PwrDriveshft"
  Speed/1 -> Transferred Power/2
  Vector Concatenate/1 -> Demux/1
  Constant1/1 -> Bus Creator5/2  "PwrDampLoss"
  Constant2/1 -> Bus Creator7/1  "PwrStoredShft"

== system CAVE_MachE_sil_test/Vehicle Under Test/Vehicle/Front Wheel Drive/Real Diff/Power Bus ==
  DriveshftTrq : Inport
  Speed : Inport  Port=2
  Bus Creator : BusCreator  Inputs=1
  Bus Creator5 : BusCreator  Inputs=2
  Bus Creator6 : BusCreator  Inputs=3
  Bus Creator7 : BusCreator  Inputs=1
  Constant : Constant  Value=0
  Constant1 : Constant  Value=0
  Constant2 : Constant  Value=0
  Demux : Demux  Outputs=3
  Power Accounting Bus Creator : autolibpowerinfoutils/Power Accounting Bus Creator  AssctBlkSelPopup=Parent reference block  RefBlkName='autolibshareddiff/Open Differential'  PwrTrnsfrdCheckBox=on  PwrNotTrnsfrdCheckBox=on  PwrStoredCheckBox=on  aMode=aMode
      settings: SourceProductName=Powertrain Blockset  SourceProductBaseCode=PW
  Signal Specification5 : SignalSpecification  Unit=W
  Transferred Power : Product
  Vector Concatenate : Concatenate  NumInputs=3
  PwrInfo : Outport
  wires:
  Bus Creator/1 -> Power Accounting Bus Creator/1
  Power Accounting Bus Creator/1 -> PwrInfo/1  "PwrInfo"
  Bus Creator5/1 -> Power Accounting Bus Creator/2
  Bus Creator6/1 -> Bus Creator/1  "PwrTrnsfrd"
  Transferred Power/1 -> Signal Specification5/1
  Signal Specification5/1 -> Vector Concatenate/3, Vector Concatenate/2, Vector Concatenate/1  "PwrDriveshft"
  Constant/1 -> Bus Creator5/1  "PwrMechLoss"
  Demux/3 -> Bus Creator6/3  "PwrAxl2"
  DriveshftTrq/1 -> Transferred Power/1
  Bus Creator7/1 -> Power Accounting Bus Creator/3
  Demux/2 -> Bus Creator6/2  "PwrAxl1"
  Demux/1 -> Bus Creator6/1  "PwrDriveshft"
  Speed/1 -> Transferred Power/2
  Vector Concatenate/1 -> Demux/1
  Constant1/1 -> Bus Creator5/2  "PwrDampLoss"
  Constant2/1 -> Bus Creator7/1  "PwrStoredShft"

== system CAVE_MachE_sil_test/Vehicle Under Test/Vehicle/Powertrain Supervisory Controller /Engine Torque Command/Accel Pedal to Traction Wheel Torque Request1 ==
  note: Convert Accelerator Pedal Position to Torque Command
      | using Motor Torque Speed Curve
  AccelPdl : Inport
  MotSpd : Inport  Port=2
  Max Motor Torque : Subsystem
  Product1 : Product
  TrqCmd : Outport  VectorParamsAs1DForOutWhenUnconnected=off
  wires:
  Max Motor Torque/1(MtrTrqMax) -> Product1/2
  MotSpd/1 -> Max Motor Torque/1(MtrSpd)
  AccelPdl/1 -> Product1/1
  Product1/1 -> TrqCmd/1

== system CAVE_MachE_sil_test/Vehicle Under Test/Vehicle/Powertrain Supervisory Controller /Engine Torque Command/Battery Management System ==
  note: Behaviorial BMS System. Limits battery charge / discharge power based on SOC.
      |
      | Charge/Discharge Limits and curves can be adjusted if using a larger battery pack
      | or motor power is changed.
  SOC : Inport
  ChrgLmt : Lookup_n-D  NumberOfTableDimensions=1  BreakpointsForDimension1=BattChargeLimitSocBpts  Table=BattChargeLimitTbl  ExtrapMethod=Clip  UseLastTableValue=on  InternalRulePriority=Speed  RndMeth=Simplest  InputSameDT=on
  DischrgLmt : Lookup_n-D  NumberOfTableDimensions=1  BreakpointsForDimension1=BattDischargeLimitSocBpts  Table=BattDischargeLimitTbl  ExtrapMethod=Clip  UseLastTableValue=on  InternalRulePriority=Speed  RndMeth=Simplest  InputSameDT=on
  MaxChrg : Constant  Value=BattChargeLimitMaxPwr
  MaxDischrg : Constant  Value=BattDischargeMaxPwr
  Product : Product
  Product1 : Product
  BattPwrDischrgLmt : Outport  VectorParamsAs1DForOutWhenUnconnected=off
  BattPwrChrgLmt : Outport  Port=2  VectorParamsAs1DForOutWhenUnconnected=off
  wires:
  DischrgLmt/1 -> Product/1
  ChrgLmt/1 -> Product1/1
  Product1/1 -> BattPwrChrgLmt/1
  Product/1 -> BattPwrDischrgLmt/1
  MaxDischrg/1 -> Product/2
  MaxChrg/1 -> Product1/2
  SOC/1 -> ChrgLmt/1, DischrgLmt/1

== system CAVE_MachE_sil_test/Vehicle Under Test/Vehicle/Powertrain Supervisory Controller /Engine Torque Command/Motor Torque Arbitration and Power Management ==
  MotTrqCmdTrac : Inport
  AccelPdl : Inport  Port=2
  BattPwrDisChrgLmt : Inport  Port=3
  "BattPwrChrgLmt " : Inport  Port=4
  MotSpd : Inport  Port=5
  MotTrqCmdRegen : Inport  Port=6
  Accel Decel Switch : Switch  Criteria=u2 > Threshold
  Compare To Constant : simulink/Logic and Bit Operations/Compare To Constant  relop=>  const=0  OutDataTypeStr=boolean
  Power Management : Subsystem
  MotTrqCmdFinal : Outport  VectorParamsAs1DForOutWhenUnconnected=off
  wires:
  Compare To Constant/1 -> Accel Decel Switch/2
  MotSpd/1 -> Power Management/3(MotSpd)
  "BattPwrChrgLmt "/1 -> Power Management/2(BattPwrChrgLmt)
  BattPwrDisChrgLmt/1 -> Power Management/1(BattPwrDischrgLmt)
  Accel Decel Switch/1 -> Power Management/4(MotTrqCmd)
  Power Management/1(MotTrqCmdFinal) -> MotTrqCmdFinal/1
  MotTrqCmdTrac/1 -> Accel Decel Switch/1
  MotTrqCmdRegen/1 -> Accel Decel Switch/3
  AccelPdl/1 -> Compare To Constant/1

== system CAVE_MachE_sil_test/Vehicle Under Test/Vehicle/Powertrain Supervisory Controller /Engine Torque Command/Series Regen Braking ==
  note: These are all torque on wheels, which is DiffRatio*torque on motor
  note: - Total brake torque request based on brake pressure and parameters of disc brakes
      | - Use as much regenerative motor braking as possible
      | - Any braking torque request that cannot be provided by the motor, will be provided by the friction brakes
  BattSoc : Inport
  VehSpd : Inport  Port=2
  MotSpd : Inport  Port=3
  "DecelCmd " : Inport  Port=4
  ChrgLmt : Lookup_n-D  NumberOfTableDimensions=1  BreakpointsForDimension1=BattChargeLimitSocBpts  Table=BattChargeLimitTbl  ExtrapMethod=Clip  UseLastTableValue=on  InternalRulePriority=Speed  RndMeth=Simplest  InputSameDT=on
  Gain : Gain  Gain=-1
  Gain1 : Gain  Gain=BrakeMaxTrq
  Gain2 : Gain  Gain=1/BrakeMaxTrq
  Max Motor Torque : LibPtSupervisoryCtrl/Powertrain Supervisory Controller /Engine Torque Command/Accel Pedal to Traction Wheel Torque Request/Max Motor Torque  SystemSampleTime=-1  Latency=0  AutoFrameSizeCalculation=off
  MinMax : MinMax  Inputs=2
  MotTrqReflectedToWheels : Gain  Gain=DiffRatio
  Product1 : Product
  Product3 : Product
  RegenBrakingCutoff : Lookup_n-D  NumberOfTableDimensions=1  BreakpointsForDimension1=SupvsryCtrlRegenSpdBpts  Table=SupvsryCtrlRegenBrkCutOffTbl  ExtrapMethod=Clip  UseLastTableValue=on  InternalRulePriority=Speed  RndMeth=Simplest  InputSameDT=on
  Saturation : Saturate  UpperLimit=1  LowerLimit=0
  Saturation1 : Saturate  UpperLimit=1  LowerLimit=0
  Subtract : Sum  Inputs=+-
  WhlTrqReflectedToMot : Gain  Gain=1/DiffRatio
  " MotTrqCmdRegen" : Outport  VectorParamsAs1DForOutWhenUnconnected=off
  " BrkCmd" : Outport  Port=2  VectorParamsAs1DForOutWhenUnconnected=off
  wires:
  Gain2/1 -> Saturation1/1  "BrkTrqReqTotal"
  Subtract/1 -> Gain2/1
  Saturation/1 -> Gain1/1
  "DecelCmd "/1 -> Saturation/1  "BrkPrsReq"
  Gain/1 -> " MotTrqCmdRegen"/1  "MotTrqCmdRegen"
  WhlTrqReflectedToMot/1 -> Gain/1
  MotTrqReflectedToWheels/1 -> MinMax/2  "MotTrqMaxWhls"
  MotSpd/1 -> Max Motor Torque/1
  BattSoc/1 -> ChrgLmt/1
  Product1/1 -> Product3/2  "RegenFactor"
  RegenBrakingCutoff/1 -> Product1/1
  VehSpd/1 -> RegenBrakingCutoff/1
  ChrgLmt/1 -> Product1/2
  MinMax/1 -> Product3/1  "min"
  Max Motor Torque/1 -> MotTrqReflectedToWheels/1  "MotTrqMax"
  Saturation1/1 -> " BrkCmd"/1
  Product3/1 -> Subtract/2, WhlTrqReflectedToMot/1  "MotTrqRegenWhl"
  Gain1/1 -> MinMax/1, Subtract/1  "BrkTrqReqTotal"

== system CAVE_MachE_sil_test/Vehicle Under Test/Vehicle/Rototest and ORNL Interface/Get Wheel Spd Cmd Based on Wheel Dynamics/WheelSpdCmd ==
  In1 : Inport
  Bus Selector : BusSelector  OutputSignals=PT IF WFL rotv,PT IF WFR rotv,PT IF WRL rotv,PT IF WRR rotv
  Mux : Mux
  Out1 : Outport
  wires:
  Mux/1 -> Out1/1
  Bus Selector/1 -> Mux/1  "<PT IF WFL rotv>"
  Bus Selector/4 -> Mux/4  "<PT IF WRR rotv>"
  In1/1 -> Bus Selector/1
  Bus Selector/3 -> Mux/3  "<PT IF WRL rotv>"
  Bus Selector/2 -> Mux/2  "<PT IF WFR rotv>"

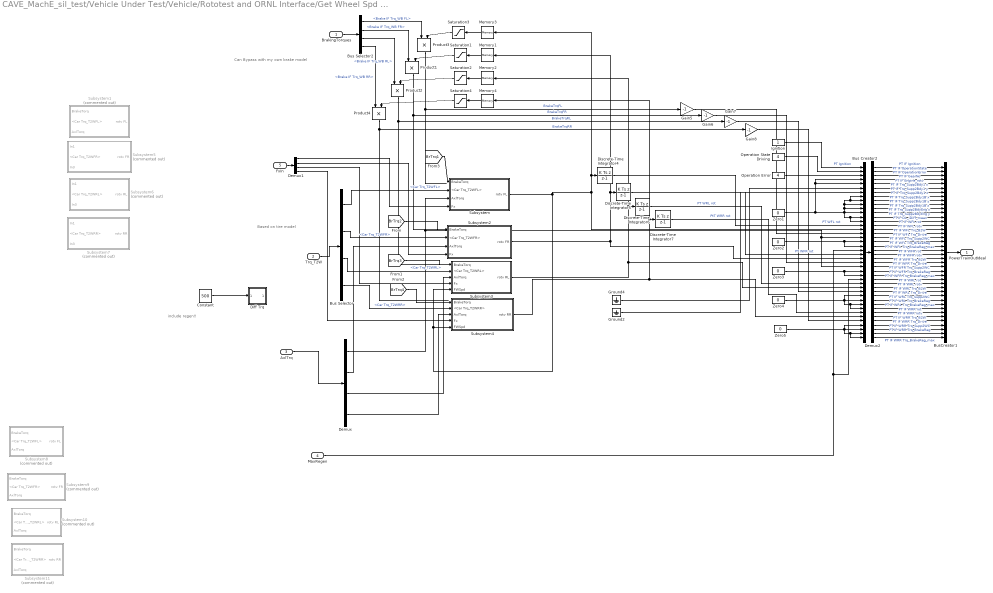
== system CAVE_MachE_sil_test/Vehicle Under Test/Vehicle/Rototest and ORNL Interface/Get Wheel Spd Cmd Based on Wheel Dynamics/Whl Dynamics & Format CM Powertrain Signal ==
  note: include regen!!
  note: Based on tire model
  note: Can Bypass with my own brake model
  BrakingTorques : Inport
  Trq_T2W : Inport  Port=2
  AxlTrq : Inport  Port=3
  MaxRegen : Inport  Port=4
  FxIn : Inport  Port=5
  Bus Creator2 : BusCreator  Inputs=42
  Bus Selector : BusSelector  OutputSignals=Car Trq_T2WFL,Car Trq_T2WFR,Car Trq_T2WRL,Car Trq_T2WRR
  Bus Selector2 : BusSelector  OutputSignals=Brake IF Trq_WB FL,Brake IF Trq_WB FR,Brake IF Trq_WB RL,Brake IF Trq_WB RR
  BusCreator1 : BusCreator  Inputs=42
  Constant : Constant  Value=500
  Demux : Demux
  Demux1 : Demux
  Demux2 : Demux  Outputs=42
  Diff Trq : Subsystem
  Discrete-Time Integrator{4..7} (4 alike) : DiscreteIntegrator  IntegratorMethod=Integration: Backward Euler  SampleTime=-1  ICPrevOutput=DiscIntNeverNeededParam  ICPrevScaledInput=DiscIntNeverNeededParam
  Gain{5..8} (4 alike) : Gain  Gain=-1
  Ground2 : Ground
  Ground4 : Ground
  Ignition : Constant
  Memory{1..4} (4 alike) : Memory
  Operation Error : Constant  Value=4
  Operation State Driving : Constant  Value=4
  Product{1..4} (4 alike) : Product  RndMeth=Zero
  Saturation{1..4} (4 alike) : Saturate  UpperLimit=1  LowerLimit=-1
  Subsystem : Subsystem
  Subsystem1 : Subsystem  Commented=on
  Subsystem10 : Subsystem  Commented=on
  Subsystem11 : Subsystem  Commented=on
  Subsystem2 : Subsystem
  Subsystem3 : Subsystem
  Subsystem4 : Subsystem
  Subsystem5 : Subsystem  Commented=on
  Subsystem6 : Subsystem  Commented=on
  Subsystem7 : Subsystem  Commented=on
  Subsystem8 : Subsystem  Commented=on
  Subsystem9 : Subsystem  Commented=on
  Zero{1..5} (5 alike) : Constant  Value=0
  PowerTrainOutIdeal : Outport
  wires:
  Saturation4/1 -> Product4/2
  Memory4/1 -> Saturation4/1
  Bus Selector2/4 -> Product4/1  "<Brake IF Trq_WB RR>"
  Product4/1 -> Gain8/1  "BrakeTrqRR"
  Saturation2/1 -> Product2/2
  Memory2/1 -> Saturation2/1
  Bus Selector2/3 -> Product2/1  "<Brake IF Trq_WB RL>"
  Product2/1 -> Gain7/1  "BrakeTrqRL"
  Saturation1/1 -> Product1/2
  Memory1/1 -> Saturation1/1
  Bus Selector2/2 -> Product1/1  "<Brake IF Trq_WB FR>"
  Product1/1 -> Gain6/1  "BrakeTrqFR"
  Memory3/1 -> Saturation3/1
  Saturation3/1 -> Product3/2
  Bus Selector2/1 -> Product3/1  "<Brake IF Trq_WB FL>"
  Product3/1 -> Gain5/1  "BrakeTrqFL"
  BrakingTorques/1 -> Bus Selector2/1
  Trq_T2W/1 -> Bus Selector/1
  Discrete-Time Integrator7/1 -> Bus Creator2/36  "PtT WRR rot"
  Discrete-Time Integrator6/1 -> Bus Creator2/29  "PT WRL rot"
  Discrete-Time Integrator5/1 -> Bus Creator2/22  "PT WFR rot"
  Discrete-Time Integrator4/1 -> Bus Creator2/15  "PT WFL rot"
  Ignition/1 -> Bus Creator2/1  "PT Ignition"
  Bus Creator2/1 -> Demux2/1
  Operation State Driving/1 -> Bus Creator2/2
  Operation Error/1 -> Bus Creator2/3
  Zero1/1 -> Bus Creator2/5, Bus Creator2/4, Bus Creator2/12, Bus Creator2/14, Bus Creator2/13, Bus Creator2/11, Bus Creator2/10, Bus Creator2/9, Bus Creator2/8
  Zero2/1 -> Bus Creator2/19, Bus Creator2/20
  Zero3/1 -> Bus Creator2/26, Bus Creator2/27
  Zero4/1 -> Bus Creator2/32, Bus Creator2/33, Bus Creator2/34, Bus Creator2/35
  Zero5/1 -> Bus Creator2/39, Bus Creator2/40, Bus Creator2/41, Bus Creator2/42
  Gain6/1 -> Bus Creator2/24
  Gain5/1 -> Bus Creator2/17
  Gain7/1 -> Bus Creator2/31
  Gain8/1 -> Bus Creator2/38
  Demux2/42 -> BusCreator1/42  "PT IF WRR Trq_BrakeReg_max"
  Demux2/41 -> BusCreator1/41  "PT IF WRR Trq_BrakeReg"
  Demux2/40 -> BusCreator1/40  "PT IF WRR Trq_Supp2WC"
  Demux2/39 -> BusCreator1/39  "PT IF WRR Trq_Drive"
  Demux2/38 -> BusCreator1/38  "PT IF WRR Trq_B2W"
  Demux2/37 -> BusCreator1/37  "PT IF WRR rotv"
  Demux2/36 -> BusCreator1/36  "PT IF WRR rot"
  Demux2/35 -> BusCreator1/35  "PT IF WRL Trq_BrakeReg_max"
  Demux2/34 -> BusCreator1/34  "PT IF WRL Trq_BrakeReg"
  Demux2/33 -> BusCreator1/33  "PT IF WRL Trq_Supp2WC"
  Demux2/32 -> BusCreator1/32  "PT IF WRL Trq_Drive"
  Demux2/31 -> BusCreator1/31  "PT IF WRL Trq_B2W"
  Demux2/30 -> BusCreator1/30  "PT IF WRL rotv"
  Demux2/29 -> BusCreator1/29  "PT IF WRL rot"
  Demux2/28 -> BusCreator1/28  "PT IF WFR Trq_BrakeReg_max"
  Demux2/27 -> BusCreator1/27  "PT IF WFR Trq_BrakeReg"
  Demux2/26 -> BusCreator1/26  "PT IF WFR Trq_Supp2WC"
  Demux2/25 -> BusCreator1/25  "PT IF WFR Trq_Drive"
  Demux2/24 -> BusCreator1/24  "PT IF WFR Trq_B2W"
  Demux2/23 -> BusCreator1/23  "PT IF WFR rotv"
  Demux2/22 -> BusCreator1/22  "PT IF WFR rot"
  Demux2/21 -> BusCreator1/21  "PT IF WFL Trq_BrakeReg_max"
  Demux2/20 -> BusCreator1/20  "PT IF WFL Trq_BrakeReg"
  Demux2/19 -> BusCreator1/19  "PT IF WFL Trq_Supp2WC"
  Demux2/18 -> BusCreator1/18  "PT IF WFL Trq_Drive"
  Demux2/17 -> BusCreator1/17  "PT IF WFL Trq_B2W"
  Demux2/16 -> BusCreator1/16  "PT IF WFL rotv"
  Demux2/15 -> BusCreator1/15  "PT IF WFL rot"
  Demux2/14 -> BusCreator1/14  "PT IF DL_iDiff_mean"
  Demux2/13 -> BusCreator1/13  "PT IF Trq_Supp2BdyEng y"
  Demux2/12 -> BusCreator1/12  "PT IF Trq_Supp2BdyEng x"
  Demux2/11 -> BusCreator1/11  "PT IF Trq_Supp2Bdy1B z"
  Demux2/10 -> BusCreator1/10  "PT IF Trq_Supp2Bdy1B y"
  Demux2/9 -> BusCreator1/9  "PT IF Trq_Supp2Bdy1B x"
  Demux2/8 -> BusCreator1/8  "PT IF Trq_Supp2Bdy1 z"
  Demux2/7 -> BusCreator1/7  "PT IF Trq_Supp2Bdy1 y"
  Demux2/6 -> BusCreator1/6  "PT IF Trq_Supp2Bdy1 x"
  Demux2/5 -> BusCreator1/5  "PT IF Engine_rotv"
  Demux2/4 -> BusCreator1/4  "PT IF GearNo"
  Demux2/3 -> BusCreator1/3  "PT IF OperationError"
  Demux2/2 -> BusCreator1/2  "PT IF OperationState"
  Demux2/1 -> BusCreator1/1  "PT IF Ignition"
  BusCreator1/1 -> PowerTrainOutIdeal/1
  Ground2/1 -> Bus Creator2/7
  Ground4/1 -> Bus Creator2/6
  Constant/1 -> Diff Trq/1(In1)
  AxlTrq/1 -> Demux/1
  Demux/1 -> Subsystem/3(AxlTorq), Bus Creator2/25, Bus Creator2/18
  MaxRegen/1 -> Bus Creator2/28, Bus Creator2/21
  Subsystem/1(rotv FL) -> Bus Creator2/16, Memory3/1, Discrete-Time Integrator4/1, Subsystem4/5(FWSpd), Subsystem3/5(FWSpd)
  Bus Selector/1 -> Subsystem/2(<Car Trq_T2WFL>)  "<Car Trq_T2WFL>"
  Subsystem2/1("rotv FR ") -> Memory1/1, Discrete-Time Integrator5/1, Bus Creator2/23
  Bus Selector/2 -> Subsystem2/2(<Car Trq_T2WFR>)  "<Car Trq_T2WFR>"
  Demux/2 -> Subsystem2/3(AxlTorq)
  Subsystem3/1(rotv RL) -> Memory2/1, Discrete-Time Integrator6/1, Bus Creator2/30
  Bus Selector/3 -> Subsystem3/2(<Car Trq_T2WRL>)  "<Car Trq_T2WRL>"
  Demux/3 -> Subsystem3/3(AxlTorq)
  Subsystem4/1(rotv RR) -> Memory4/1, Discrete-Time Integrator7/1, Bus Creator2/37
  Bus Selector/4 -> Subsystem4/2(<Car Trq_T2WRR>)  "<Car Trq_T2WRR>"
  Demux/4 -> Subsystem4/3(AxlTorq)
  FxIn/1 -> Demux1/1
  Demux1/1 -> Subsystem/4(Fx)
  Demux1/2 -> Subsystem2/4(Fx)
  Demux1/3 -> Subsystem3/4(Fx)
  Demux1/4 -> Subsystem4/4(Fx)
  [BrTrq4] -> Subsystem4/1(BrakeTorq)
  [BrTrq3] -> Subsystem3/1(BrakeTorq)
  [BrTrq2] -> Subsystem2/1(BrakeTorq)
  [BrTrq1] -> Subsystem/1(BrakeTorq)

== system CAVE_MachE_sil_test/Vehicle Under Test/Vehicle/Rototest and ORNL Interface/To Rototest with Band-Aid/Band-Aid ==
  InSpd_rpm : Inport
  InTrq_Nm : Inport  Port=2
  BRAKE_PRESSED : Inport  Port=3
  VehSpd_kph : Inport  Port=4
  Band-Aid : Stateflow chart  BlockKeywords=__PRM__SERIALIZED__DATA__:Stateflow Chart,Stateflow Diagram  TreatAsAtomicUnit=on
  BrkLatchThr_Nm : Constant  Value=-50
  Header : VSIGenLib/Header  not=''
  LaunchSpdThr_rpm : Constant  Value=2
  LaunchTrqThr_Nm : Constant  Value=20
  SettleTime_s : Constant  Value=5
  SpdLatchThr_rpm : Constant  Value=1e-5
  Terminator : Terminator
  Terminator1 : Terminator
  VehSpdThr_kph : Constant  Value=0.2
  dStop : Constant  Value=0
  OutMode : Outport
  OutSpd_rpm : Outport  Port=2
  tag scope: Mode=global
  wires:
  InSpd_rpm/1 -> Band-Aid/5(InSpd)  "InSpd_rpm"
  LaunchTrqThr_Nm/1 -> Band-Aid/2(LaunchTrqThr)
  SpdLatchThr_rpm/1 -> Band-Aid/3(SpdLatchThr)
  Band-Aid/3(State) -> Terminator/1  "State"
  LaunchSpdThr_rpm/1 -> Band-Aid/1(LaunchSpdThr)
  SettleTime_s/1 -> Band-Aid/7(SettleTime)
  Band-Aid/1(OutMode) -> [Mode], OutMode/1  "OutMode"
  BrkLatchThr_Nm/1 -> Terminator1/1
  Band-Aid/2(OutSpd) -> OutSpd_rpm/1  "OutSpd"
  InTrq_Nm/1 -> Band-Aid/6(InTrq)  "InTrq_Nm"
  dStop/1 -> Band-Aid/8(dStop)
  BRAKE_PRESSED/1 -> Band-Aid/4(BrkSw)
  VehSpd_kph/1 -> Band-Aid/9(VehSpd_kph)  "VehicleSpeed_kph"
  VehSpdThr_kph/1 -> Band-Aid/10(VehSpdThr_kph)
